simulink model "model_teste"  (R2020a)
settings: Solver=VariableStepAuto  StartTime=0.0  StopTime=10.0  RelTol=1e-3
values from neighbouring files (symbols this model uses):
  x = [-0.85 -0.86 -0.87 -0.99 -1.1 -1.15 -1.23 -1.34 -1.45 -1.54 -1.61 -1.68 ... (7634 elements, 1x7634)]    [ss60.mat]    (also in z_get_y_from_x.m = Bezier.get_x3_from_y(C, y); z_rational.m = P(:,1); z_untitled.m = r.alc/1000.)
  y = [97.48 98.87 100.19 100.56 100.92 101.31 102.85 104.32 105.96 107.45 109.56 111.05 ... (7634 elements, 1x7634)]    [ss60.mat]    (also in z_get_y_from_x.m = 2.1; z_rational.m = P(:,2); z_untitled.m = r.h/1000.; zz_model.m = Bez.get_P_from_x(C, 40))
settings Model: Creator=Daniel  LastModifiedBy=Daniel

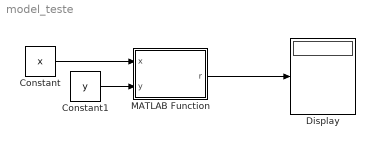
== system model_teste ==
  Constant : Constant  Value=x
  Constant1 : Constant  Value=y
  Display : Display
  MATLAB Function : MATLAB Function  TreatAsAtomicUnit=on
  wires:
  MATLAB Function/1(r) -> Display/1
  Constant/1 -> MATLAB Function/1(x)
  Constant1/1 -> MATLAB Function/2(y)

== matlab function model_teste/MATLAB Function ==
  data: r output; x input; y input
function r = fcn(x, y)

    r = zz_model(x, y);
    
end
